simulink subsystem "PersecucionPura"  (R2023b)
settings: Solver=VariableStepAuto  StartTime=0.0  StopTime=10.0  RelTol=1e-3
libraries: robotalgslib x1
settings Model: Creator=pablo  LastModifiedBy=pablo

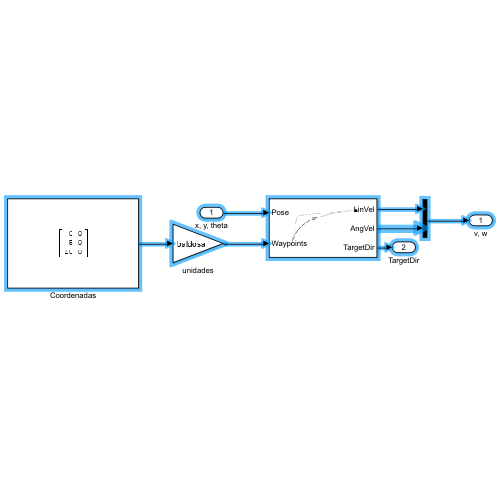
[thumbnail: Simulink's stored preview of the top-level diagram]
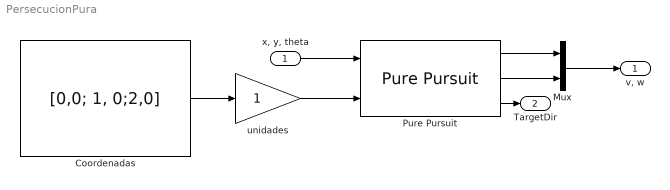
== system PersecucionPura ==
  "x, y, theta" : Inport
  Coordenadas : Constant  Value=[0,0; 1, 0;2,0]
  Mux : Mux  Inputs=2
  Pure Pursuit : robotalgslib/Pure Pursuit  DesiredLinearVelocity=0.205  MaxAngularVelocity=1.5  LookaheadDistance=0.05  TargetDirPort=on  SimulateUsing=Code generation
      settings: LibrarySourceBlock=navlib/Control Algorithms/Pure Pursuit
  unidades : Gain
  "v, w" : Outport
  TargetDir : Outport  Port=2
  wires:
  Pure Pursuit/3 -> TargetDir/1
  "x, y, theta"/1 -> Pure Pursuit/1
  Coordenadas/1 -> unidades/1
  Pure Pursuit/1 -> Mux/1
  Mux/1 -> "v, w"/1
  unidades/1 -> Pure Pursuit/2
  Pure Pursuit/2 -> Mux/2
